simulink model "chap1_5"  (Simulink 3.00)
settings: Solver=ode4  StartTime=0.0  StopTime=2  RelTol=1e-3
settings Model: SaveTime=off  SaveOutput=off  Decimation=100

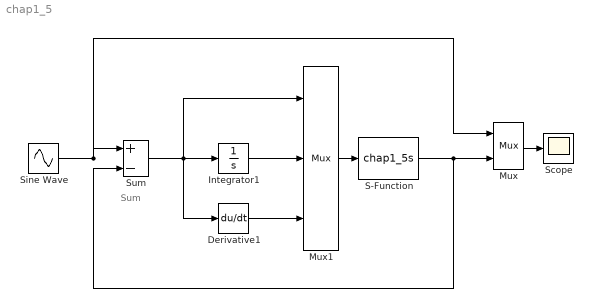
== system chap1_5 ==
  note: Sum
  Derivative1 : Derivative
  Integrator1 : Integrator  ExternalReset=none  InitialConditionSource=internal  InitialCondition=0  LimitOutput=off  UpperSaturationLimit=inf  LowerSaturationLimit=-inf  ShowSaturationPort=off  ShowStatePort=off  AbsoluteTolerance=auto
  Mux : Mux  Inputs=2
      settings: DisplayOption=none
  Mux1 : Mux  Inputs=3
      settings: DisplayOption=none
  S-Function : S-Function  FunctionName=chap1_5s  PortCounts=[]  SFunctionModules=''
  Scope : Scope
      settings: TimeRange=0.2  YMin=-0.051  YMax=-0.041  SaveToWorkspace=off  SaveName=ScopeData  MaxRows=50000  Decimation=0.001  SampleInput=on  SampleTime=0.001
  Sine Wave : Sin  Amplitude=0.50  Frequency=1*2*pi  Phase=0  SampleTime=0
  Sum : Sum  Inputs=|+-  SaturateOnIntegerOverflow=on
  wires:
  Mux/1 -> Scope/1
  S-Function/1 -> Mux/2, Sum/2
  Mux1/1 -> S-Function/1
  Sine Wave/1 -> Sum/1, Mux/1
  Derivative1/1 -> Mux1/3
  Integrator1/1 -> Mux1/2
  Sum/1 -> Integrator1/1, Derivative1/1, Mux1/1
